simulink model "driver_model_replanning_R1"  (R2023b)
settings: Solver=VariableStepAuto  StartTime=0.0  StopTime=50  RelTol=1e-3
libraries: slpidlib x2, Solver_SF x1
settings Model: DataTypeOverride=Double  MinMaxOverflowLogging=ForceOff  Creator=황수빈  LastModifiedBy=황수빈

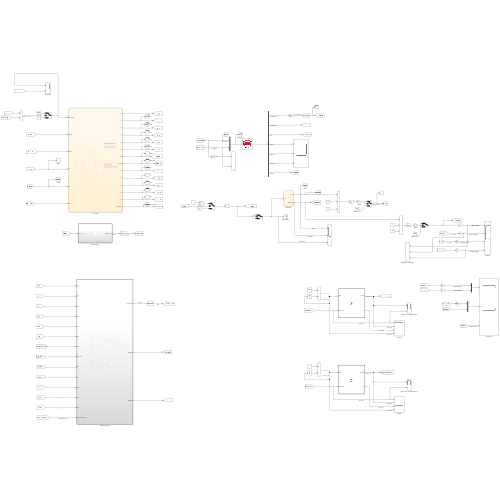
[thumbnail: Simulink's stored preview of the top-level diagram]
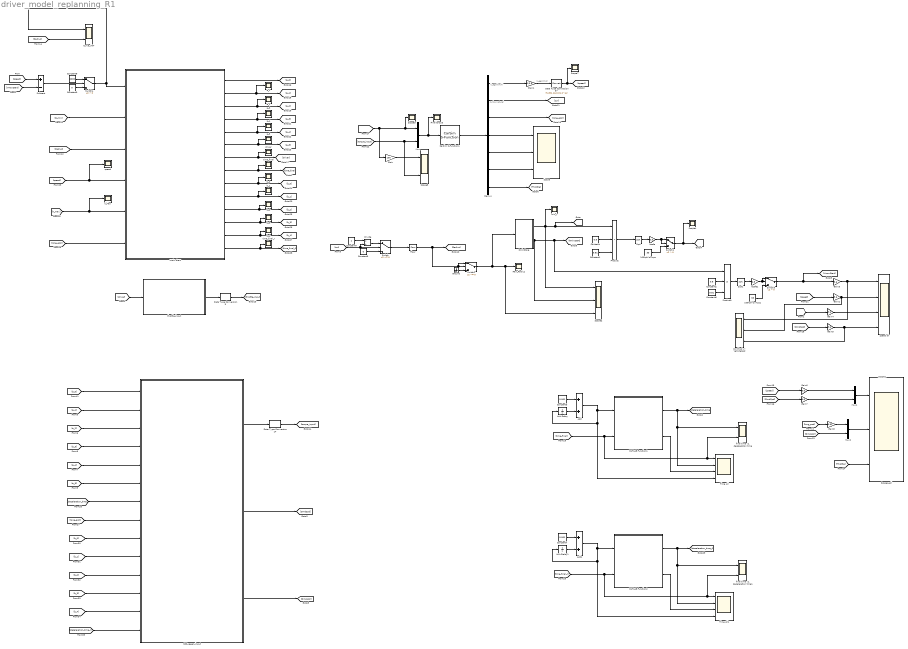
== system driver_model_replanning_R1 ==
  note: V_ego(m/s)
  note: V_ego(km/h)
  note: cur(curvature)
  100kph to mps : Constant  Value=33
  100kph to mps1 : Constant  Value=33
  Add : Sum
  Add1 : Sum
  CarSim S-Function1 : Solver_SF/CarSim S-Function  Priority=1  SIMFILE=simfile.sim  Run_RTs=off  vs_state_ind=Run  StopMode_ind=Vehicle Model
  Constant : Constant  Value=0.8
  Constant1 : Constant  Value=9.81
  Constant2 : Constant  Value=0.8
  Constant3 : Constant  Value=0.001
  Constant4 : Constant
  Constant5 : Constant  Value=0
  Constant6 : Constant  Value=9.81
  Constant7 : Constant  Value=0.001
  Constant8 : Constant  Value=2000
  Constant9 : Constant  Value=0
  Curve_INIT : Scope  NumInputPorts=2
  Data Type Conversion14 : DataTypeConversion  OutDataTypeStr=fixdt(1,16,0)  RndMeth=Nearest  SaturateOnIntegerOverflow=off
  Data Type Conversion3 : DataTypeConversion  OutDataTypeStr=fixdt(1,16,0)  RndMeth=Nearest  SaturateOnIntegerOverflow=off
  Data Type Conversion37 : DataTypeConversion  OutDataTypeStr=fixdt(1,16,0.01,2^-6)  RndMeth=Simplest  SaturateOnIntegerOverflow=off
  Demux : Demux  Outputs=7
  Divide : Product  Inputs=*/
  DmdSpd vs VehicleSpd : Scope  NumInputPorts=3
  Final torque : Scope
  Floor : Rounding
  Gain : Gain  Gain=100
  Gain1 : Gain  Gain=1/3.6
  Gain{2..7} (6 alike) : Gain  Gain=3.6
  Gain8 : Gain  Gain=9.81
  Ground : Ground
  MATLAB Function1 : MATLAB Function  TreatAsAtomicUnit=on
  MATLAB Function2 : MATLAB Function  TreatAsAtomicUnit=on
  Mux : Mux  Inputs=2
  Mux1 : Mux  Inputs=2
  Mux2 : Mux  Inputs=2
  Nsafe : Gain  Gain=0.5
  Nsafe1 : Gain  Gain=0.5
  Product : Product  Inputs=3
  Product1 : Product  Inputs=3
  Raw_Radius : Scope
  RminStore : Stateflow chart  TreatAsAtomicUnit=on
  SRS_regen_input : Subsystem  TreatAsAtomicUnit=on
  Scope : Scope  NumInputPorts=3
  Scope{1,3..4,7} (4 alike) : Scope
  Scope2 : Scope  NumInputPorts=3
  Scope5 : Scope  NumInputPorts=2
  Scopes_all : Scope  NumInputPorts=3
  Sqrt : Sqrt
  Sqrt1 : Sqrt
  Subtract : Sum  Inputs=+-
  Switch : Switch  Criteria=u2 ~= 0  SaturateOnIntegerOverflow=off  InputSameDT=off
  Switch1 : Switch  Criteria=u2 > Threshold  SaturateOnIntegerOverflow=off  InputSameDT=off
  Switch2 : Switch  Criteria=u2 ~= 0  SaturateOnIntegerOverflow=off  InputSameDT=off
  Switch3 : Switch  Criteria=u2 > Threshold  SaturateOnIntegerOverflow=off  InputSameDT=off
  Switch4 : Switch  Criteria=u2 > Threshold  SaturateOnIntegerOverflow=off  InputSameDT=off
  Time All : Scope  NumInputPorts=4
  Time All1 : Scope  NumInputPorts=4
  Unit Delay : UnitDelay  SampleTime=-1  HasFrameUpgradeWarning=on
  Unit Delay1 : UnitDelay  SampleTime=-1  HasFrameUpgradeWarning=on
  V_Max : Scope
  a_{1..5} (5 alike) : Scope
  b_{0..4} (5 alike) : Scope
  driver : Scope
  final time vs. deceleration time : Scope  NumInputPorts=2
  final time vs. deceleration time1 : Scope  NumInputPorts=2
  main chart : Stateflow chart  TreatAsAtomicUnit=on
  min_r : Scope
  speed : Scope
  speed all : Scope  NumInputPorts=4
  throttle_input : Subsystem  TreatAsAtomicUnit=on  SystemSampleTime=0.01
  time_final : Scope
  time_final_r : Scope
  wires:
  [a_4] -> SRS_regen_input/5(a_4)
  [speed] -> Gain2/1  "m/s -> kph"
  100kph to mps/1 -> Switch1/3
  [a_3] -> SRS_regen_input/4(a_3)
  Gain/1 -> Scope5/1
  [Throttle] -> Scopes_all/3  "Throttle Pressure"
  Gain7/1 -> Mux1/2  "TARGET SPEED"
  Floor/1 -> Switch2/1, Switch2/2, [Radius]
  [DmdSpd] -> Gain7/1
  [DmdAccl] -> Mux2/2
  Sqrt1/1 -> Nsafe1/1
  [deceleration_time] -> SRS_regen_input/7(time t)
  Gain6/1 -> Mux1/1  "VEHICLE SPEED"
  Mux2/1 -> Scopes_all/2
  Demux/2 -> [cur]
  Product1/1 -> Sqrt1/1
  Gain8/1 -> Mux2/1
  Gain5/1 -> DmdSpd vs VehicleSpd/3, speed all/4  "DEMAND SPEED"
  Mux1/1 -> Scopes_all/1
  Add/1 -> Unit Delay/1, Time All/4, MATLAB Function1/1(time)  "current_time"
  [long_accl] -> Gain8/1
  Demux/5 -> Scope/2  "M_Mtr_D2"
  Demux/7 -> [Throttle]  "Thrtl_SC"
  Nsafe/1 -> Switch1/1, Switch1/2
  SRS_regen_input/3(DmdAccl) -> [DmdAccl]
  [speed] -> Gain6/1
  SRS_regen_input/2(DmdSpd) -> [DmdSpd]
  Switch3/1 -> [VmaxStart], Gain3/1
  100kph to mps1/1 -> Switch3/3
  MATLAB Function1/1(t_output) -> [deceleration_time], final time vs. deceleration time/1, Time All/2  "decel_time"
  [Radius] -> main chart/3(radius)
  main chart/4(a_3) -> a_3/1, [a_3]
  [DmdSpd] -> Gain5/1
  Demux/6 -> Scope/3  "PwMtC_D2"
  [V_max] -> Gain4/1  "m/s -> kph"
  [a_2] -> SRS_regen_input/3(a_2)
  Demux/1 -> Gain1/1
  Gain4/1 -> speed all/3  "TARGET SPEED2"
  Constant2/1 -> Product1/2
  Unit Delay/1 -> Add/2
  Demux/4 -> Scope/1  "M_Mt_D2"
  Gain3/1 -> DmdSpd vs VehicleSpd/1, speed all/1  "TARGET SPEED"
  Nsafe1/1 -> Switch3/1, Switch3/2
  [Radius] -> Curve_INIT/2
  Product/1 -> Sqrt/1
  main chart/5(a_4) -> [a_4], a_4/1
  [speed] -> speed/1, main chart/4(v0)
  RminStore/1(Rmin) -> min_r/1, [R_min], Product/1, Scope2/1  "minR"
  Switch2/1 -> Scope2/3, Raw_Radius/1, RminStore/1(r)  "Raw Radius"
  [long_accl] -> SRS_regen_input/8(long. accl)
  [throttle_input] -> Mux/1, Scope3/1, Gain/1  "throttle input"
  Sqrt/1 -> Nsafe/1
  [torque_input] -> Scope5/2, Mux/2  "torque input"
  Ground/1 -> Switch2/3
  Gain1/1 -> Data Type Conversion37/1
  [a_5] -> SRS_regen_input/6(a_5)
  [time_final] -> MATLAB Function1/2(time_final), final time vs. deceleration time/2, Time All/1  "time_final"
  [long_accl] -> main chart/6(a0)
  [R_min] -> main chart/2(R_min)
  Constant3/1 -> Add/1
  Constant9/1 -> Switch4/3
  throttle_input/1(throttle_input) -> Data Type Conversion3/1  "before"
  Constant/1 -> Product/2
  Switch4/1 -> main chart/1(Curve_INIT), Curve_INIT/1
  Subtract/1 -> Switch4/2  "speed > v_max"
  [V_max] -> V_Max/1, main chart/5(vf)
  MATLAB Function1/2(p) -> Time All/3  "prev_time"
  [VmaxStart] -> Subtract/2
  [a_1] -> SRS_regen_input/2(a_1)
  main chart/2(a_1) -> a_1/1, [a_1]
  main chart/3(a_2) -> a_2/1, [a_2]
  main chart/6(a_5) -> [a_5], a_5/1
  [a_0] -> SRS_regen_input/1(a_0)
  Constant8/1 -> Switch4/1
  Mux/1 -> CarSim S-Function1/1, Final torque/1
  Data Type Conversion3/1 -> [throttle_input]  "after"
  main chart/7(driver) -> [driver], driver/1
  Data Type Conversion37/1 -> Scope7/1, [speed]
  Demux/3 -> [long_accl]  "accel"
  Divide/1 -> Switch/1
  [cur] -> Switch/2, Divide/2
  RminStore/2(RminStart) -> Scope2/2, [RminStart], Product1/1  "minR Start"
  main chart/8(time_final) -> [time_final], time_final/1
  Switch/1 -> Floor/1
  Gain2/1 -> DmdSpd vs VehicleSpd/2, speed all/2  "VEHICLE SPEED"
  [driver] -> throttle_input/1(driver)
  main chart/1(a_0) -> [a_0]
  Constant6/1 -> Product1/3
  Constant1/1 -> Product/3
  Constant4/1 -> Divide/1
  Data Type Conversion14/1 -> [torque_input]  "after"
  [speed] -> Subtract/1
  SRS_regen_input/1(torque_input) -> Data Type Conversion14/1  "before"
  Constant5/1 -> Switch/3
  CarSim S-Function1/1 -> Demux/1
  Switch1/1 -> Scope4/1, [V_max]  "target speed(m/s)"
  main chart/9(b_0) -> b_0/1, [b_0]
  main chart/10(b_1) -> b_1/1, [b_1]
  main chart/11(b_2) -> b_2/1, [b_2]
  main chart/12(b_3) -> b_3/1, [b_3]
  main chart/13(b_4) -> b_4/1, [b_4]
  main chart/14(time_final_r) -> time_final_r/1, [time_final_r]
  [b_0] -> SRS_regen_input/9(b_0)
  [b_1] -> SRS_regen_input/10(b_1)
  [b_2] -> SRS_regen_input/11(b_2)
  [b_3] -> SRS_regen_input/12(b_3)  "b_3"
  [b_4] -> SRS_regen_input/13(b_4)  "b_4"
  [time_final_r] -> MATLAB Function2/2(time_final_r), final time vs. deceleration time1/2, Time All1/1  "time_final"
  MATLAB Function2/1(t_output2) -> [deceleration_time_r], final time vs. deceleration time1/1, Time All1/2  "decel_time"
  Unit Delay1/1 -> Add1/2
  Constant7/1 -> Add1/1
  MATLAB Function2/2(p2) -> Time All1/3  "prev_time"
  Add1/1 -> Unit Delay1/1, Time All1/4, MATLAB Function2/1(time)  "current_time"
  [deceleration_time_r] -> SRS_regen_input/14(deceleration_time_r)  "deceleration_time_r"

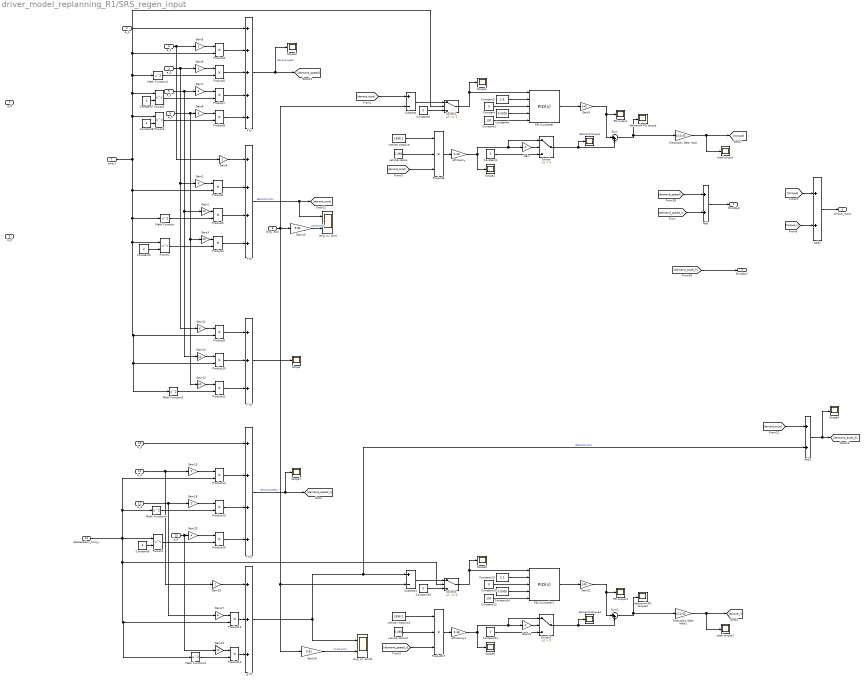
== system driver_model_replanning_R1/SRS_regen_input ==
  a_0 : Inport
  a_1 : Inport  Port=2
  a_2 : Inport  Port=3
  a_3 : Inport  Port=4
  a_4 : Inport  Port=5
  a_5 : Inport  Port=6
  time t : Inport  Port=7
  long. accl : Inport  Port=8
  b_0 : Inport  Port=9
  b_1 : Inport  Port=10
  b_2 : Inport  Port=11
  b_3 : Inport  Port=12
  b_4 : Inport  Port=13
  deceleration_time_r : Inport  Port=14
  Add : Sum
  Add1 : Sum
  Add2 : Sum
  Constant{,1,6,10..11,15} (6 alike) : Constant  Value=0
  Constant12 : Constant  Value=100
  Constant13 : Constant  Value=2.2
  Constant14 : Constant  Value=0.0005
  Constant2 : Constant  Value=100
  Constant3 : Constant  Value=2.8
  Constant4 : Constant  Value=0.0005
  Constant5 : Constant  Value=3
  Constant7 : Constant  Value=3
  Constant8 : Constant  Value=4
  Constant9 : Constant  Value=3
  Gain : Gain  Gain=-1
  Gain1 : Gain  Gain=12
  Gain10 : Gain  Gain=24
  Gain11 : Gain  Gain=6
  Gain12 : Gain  Gain=60
  Gain{4..5,13,19} (4 alike) : Gain  Gain=2
  Gain14 : Gain  Gain=12
  Gain15 : Gain  Gain=9.81
  Gain16 : Gain  Gain=9.81
  Gain17 : Gain  Gain=6
  Gain18 : Gain  Gain=3
  Gain2 : Gain  Gain=6
  Gain20 : Gain  Gain=4
  Gain21 : Gain  Gain=-1
  Gain22 : Gain  Gain=245
  Gain3 : Gain  Gain=20
  Gain6 : Gain  Gain=3
  Gain7 : Gain  Gain=4
  Gain8 : Gain  Gain=5
  Gain9 : Gain  Gain=245
  Math Function{,1..4} (5 alike) : Math  Operator=square
  PD output : Scope
  PD output1 : Scope
  PID Controller : slpidlib/PID Controller  Controller=PID  Form=Parallel  TimeDomain=Continuous-time  UseExternalTs=off  SampleTime=-1  IntegratorMethod=Forward Euler  FilterMethod=Forward Euler  ControllerParametersSource=external  P=1  I=1  UseKiTs=off  D=0  N=100  UseFilter=on  TunerSelectOption=Transfer Function Based (PID Tuner App)  InitialConditionSource=internal  InitialConditionForIntegrator=0  InitialConditionForFilter=0  DifferentiatorICPrevScaledInput=0  ExternalReset=none  TrackingMode=off  Kt=1  LimitOutput=off  SatLimitsSource=internal  UpperSaturationLimit=inf  LowerSaturationLimit=-inf  LinearizeAsGain=on  AntiWindupMode=none  Kb=1  LimitIntegrator=off  UpperIntegratorSaturationLimit=inf  LowerIntegratorSaturationLimit=-inf  POutMin=[]  POutMax=[]  IOutMin=[]  IOutMax=[]  DOutMin=[]  DOutMax=[]  NOutMin=[]  NOutMax=[]  SumOutMin=[]  SumOutMax=[]  SaturationOutMin=[]  SaturationOutMax=[]  PParamMin=[]  PParamMax=[]  IParamMin=[]  IParamMax=[]  DParamMin=[]  DParamMax=[]  NParamMin=[]  NParamMax=[]  KbParamMin=[]  KbParamMax=[]  KtParamMin=[]  KtParamMax=[]  KbOutMin=[]  KbOutMax=[]  KtOutMin=[]  KtOutMax=[]  IntegratorOutMin=[]  IntegratorOutMax=[]  FilterOutMin=[]  FilterOutMax=[]  SumI1OutMin=[]  SumI1OutMax=[]  SumI2OutMin=[]  SumI2OutMax=[]  SumI3OutMin=[]  SumI3OutMax=[]  SumI4OutMin=[]  SumI4OutMax=[]  SumDOutMin=[]  SumDOutMax=[]  DifferentiatorOutMin=[]  DifferentiatorOutMax=[]  FilterDiffOutCoefMin=[]  FilterDiffOutCoefMax=[]  ReciprocalOutMin=[]  ReciprocalOutMax=[]  SumDenOutMin=[]  SumDenOutMax=[]  SumNumOutMin=[]  SumNumOutMax=[]  DivideOutMin=[]  DivideOutMax=[]  UdiffTsProdOutMin=[]  UdiffTsProdOutMax=[]  NTsProdOutMin=[]  NTsProdOutMax=[]  UintegralTsProdOutMin=[]  UintegralTsProdOutMax=[]  UngainTsProdOutMin=[]  UngainTsProdOutMax=[]  ClampingZeroOutDataTypeStr=Inherit: Inherit via back propagation  ClampingZeroOutMin=[]  ClampingZeroOutMax=[]  FilterDenConstantOutDataTypeStr=Inherit: Inherit via back propagation  FilterDenConstantOutMin=[]  FilterDenConstantOutMax=[]  PCopyOutDataTypeStr=Inherit: Inherit via back propagation  PCopyOutMin=[]  PCopyOutMax=[]  NCopyOutDataTypeStr=Inherit: Inherit via back propagation  NCopyOutMin=[]  NCopyOutMax=[]  IntegratorContinuousStateAttributes=''  IntegratorStateMustResolveToSignalObject=off  IntegratorRTWStateStorageClass=Auto  FilterContinuousStateAttributes=''  FilterStateMustResolveToSignalObject=off  FilterRTWStateStorageClass=Auto  ParallelPVariant=ExternalParameters  IdealPVariant=Disabled  IVariant=ExternalParameters  DVariant=ExternalParameters  IntegratorVariant=Continuous  SatVariant=Disabled  AWVariant=Passthrough  PCopyVariant=Disabled  TRVariant=Disabled  FdbkBlocksVariant=Forward  IdealPFdbkVariant=Disabled  SatFdbkVariant=Disabled  DerivativeFilterVariant=ContFilter  NVariant=ExternalParameters  NCopyVariant=Disabled  FilterICVariant=InternalICsFilter  IntegratorICVariant=InternalICs  ExternalResetVariant=Disabled  TRSumVariant=Passthrough  SumFdbkVariant=Disabled  SumVariant=Sum_PID  TsampFilterVariant=InternalTs  TsampNgainVariant=Passthrough  TsampIntegralVariant=Disabled_SignalSpec  ExternalSaturationOutDataTypeStr=Inherit: Same as second input
  PID Controller1 : slpidlib/PID Controller  Controller=PID  Form=Parallel  TimeDomain=Continuous-time  UseExternalTs=off  SampleTime=-1  IntegratorMethod=Forward Euler  FilterMethod=Forward Euler  ControllerParametersSource=external  P=1  I=1  UseKiTs=off  D=0  N=100  UseFilter=on  TunerSelectOption=Transfer Function Based (PID Tuner App)  InitialConditionSource=internal  InitialConditionForIntegrator=0  InitialConditionForFilter=0  DifferentiatorICPrevScaledInput=0  ExternalReset=none  TrackingMode=off  Kt=1  LimitOutput=off  SatLimitsSource=internal  UpperSaturationLimit=inf  LowerSaturationLimit=-inf  LinearizeAsGain=on  AntiWindupMode=none  Kb=1  LimitIntegrator=off  UpperIntegratorSaturationLimit=inf  LowerIntegratorSaturationLimit=-inf  POutMin=[]  POutMax=[]  IOutMin=[]  IOutMax=[]  DOutMin=[]  DOutMax=[]  NOutMin=[]  NOutMax=[]  SumOutMin=[]  SumOutMax=[]  SaturationOutMin=[]  SaturationOutMax=[]  PParamMin=[]  PParamMax=[]  IParamMin=[]  IParamMax=[]  DParamMin=[]  DParamMax=[]  NParamMin=[]  NParamMax=[]  KbParamMin=[]  KbParamMax=[]  KtParamMin=[]  KtParamMax=[]  KbOutMin=[]  KbOutMax=[]  KtOutMin=[]  KtOutMax=[]  IntegratorOutMin=[]  IntegratorOutMax=[]  FilterOutMin=[]  FilterOutMax=[]  SumI1OutMin=[]  SumI1OutMax=[]  SumI2OutMin=[]  SumI2OutMax=[]  SumI3OutMin=[]  SumI3OutMax=[]  SumI4OutMin=[]  SumI4OutMax=[]  SumDOutMin=[]  SumDOutMax=[]  DifferentiatorOutMin=[]  DifferentiatorOutMax=[]  FilterDiffOutCoefMin=[]  FilterDiffOutCoefMax=[]  ReciprocalOutMin=[]  ReciprocalOutMax=[]  SumDenOutMin=[]  SumDenOutMax=[]  SumNumOutMin=[]  SumNumOutMax=[]  DivideOutMin=[]  DivideOutMax=[]  UdiffTsProdOutMin=[]  UdiffTsProdOutMax=[]  NTsProdOutMin=[]  NTsProdOutMax=[]  UintegralTsProdOutMin=[]  UintegralTsProdOutMax=[]  UngainTsProdOutMin=[]  UngainTsProdOutMax=[]  ClampingZeroOutDataTypeStr=Inherit: Inherit via back propagation  ClampingZeroOutMin=[]  ClampingZeroOutMax=[]  FilterDenConstantOutDataTypeStr=Inherit: Inherit via back propagation  FilterDenConstantOutMin=[]  FilterDenConstantOutMax=[]  PCopyOutDataTypeStr=Inherit: Inherit via back propagation  PCopyOutMin=[]  PCopyOutMax=[]  NCopyOutDataTypeStr=Inherit: Inherit via back propagation  NCopyOutMin=[]  NCopyOutMax=[]  IntegratorContinuousStateAttributes=''  IntegratorStateMustResolveToSignalObject=off  IntegratorRTWStateStorageClass=Auto  FilterContinuousStateAttributes=''  FilterStateMustResolveToSignalObject=off  FilterRTWStateStorageClass=Auto  ParallelPVariant=ExternalParameters  IdealPVariant=Disabled  IVariant=ExternalParameters  DVariant=ExternalParameters  IntegratorVariant=Continuous  SatVariant=Disabled  AWVariant=Passthrough  PCopyVariant=Disabled  TRVariant=Disabled  FdbkBlocksVariant=Forward  IdealPFdbkVariant=Disabled  SatFdbkVariant=Disabled  DerivativeFilterVariant=ContFilter  NVariant=ExternalParameters  NCopyVariant=Disabled  FilterICVariant=InternalICsFilter  IntegratorICVariant=InternalICs  ExternalResetVariant=Disabled  TRSumVariant=Passthrough  SumFdbkVariant=Disabled  SumVariant=Sum_PID  TsampFilterVariant=InternalTs  TsampNgainVariant=Passthrough  TsampIntegralVariant=Disabled_SignalSpec  ExternalSaturationOutDataTypeStr=Inherit: Same as second input
  Power{1..4} (4 alike) : Math  Operator=pow
  Product{1..5,7..16} (15 alike) : Product
  Product17 : Product  Inputs=3
  Product6 : Product  Inputs=3
  Reduction Gear ratio : Gain  Gain=1/10.65
  Reduction Gear ratio1 : Gain  Gain=1/10.65
  Scope{,1..7} (8 alike) : Scope
  Subtract : Sum  Inputs=+-
  Subtract1 : Sum  Inputs=+-
  Sum : Sum  Inputs=|++
  Sum1 : Sum  Inputs=|++
  Switch : Switch  Criteria=u2 > Threshold  SaturateOnIntegerOverflow=off  InputSameDT=off
  Switch1 : Switch  Criteria=u2 ~= 0  SaturateOnIntegerOverflow=off  InputSameDT=off
  Switch2 : Switch  Criteria=u2 > Threshold  SaturateOnIntegerOverflow=off  InputSameDT=off
  Switch3 : Switch  Criteria=u2 ~= 0  SaturateOnIntegerOverflow=off  InputSameDT=off
  demand torque : Scope
  demand torque1 : Scope
  demand+PD torque : Scope
  demand+PD torque1 : Scope
  efficiency : Gain  Gain=0.46
  efficiency1 : Gain  Gain=0.46
  f'''(t) : Sum  Inputs=+++
  f''(t) : Sum  Inputs=4
  f'(t) : Sum  Inputs=5
  f'(t)1 : Sum  Inputs=4
  g''(t) : Sum  Inputs=3
  long vs. dmd : Scope  NumInputPorts=2
  long vs. dmd1 : Scope  NumInputPorts=2
  total torque : Scope
  total torque1 : Scope
  vehicle massive : Constant  Value=1898.2
  vehicle massive1 : Constant  Value=1898.2
  vehicle radius : Constant  Value=0.468
  vehicle radius1 : Constant  Value=0.468
  torque_input : Outport
  DmdSpd : Outport  Port=2
  DmdAccl : Outport  Port=3
  wires:
  Constant5/1 -> Power1/2
  Product2/1 -> f''(t)/3
  Product4/1 -> f''(t)/4
  Power1/1 -> Product4/2
  Math Function/1 -> Product2/2
  Product6/1 -> efficiency/1
  efficiency/1 -> Scope2/1, Switch/1, Gain/1
  Constant1/1 -> Switch/3
  Gain/1 -> Switch/2
  f''(t)/1 -> long vs. dmd/1, [demand_accel]  "DEMAND ACCL"
  Gain1/1 -> Product2/1
  Gain3/1 -> Product4/1
  Gain4/1 -> f''(t)/1
  Gain2/1 -> Product1/1
  Product1/1 -> f''(t)/2
  Subtract/1 -> Switch1/1
  Switch1/1 -> PID Controller/1, Scope1/1
  Constant6/1 -> Switch1/3
  Constant2/1 -> PID Controller/5
  Constant4/1 -> PID Controller/4
  Constant/1 -> PID Controller/3
  Constant3/1 -> PID Controller/2
  PID Controller/1 -> Gain9/1
  Product3/1 -> f'(t)/2
  Product5/1 -> f'(t)/3
  Product7/1 -> f'(t)/4
  Product8/1 -> f'(t)/5
  Gain5/1 -> Product3/1
  Gain6/1 -> Product5/1
  Gain7/1 -> Product7/1
  Gain8/1 -> Product8/1
  f'(t)/1 -> Scope3/1, [demand_speed]  "demand speed"
  Math Function1/1 -> Product5/2
  Power2/1 -> Product7/2
  Power3/1 -> Product8/2
  Constant7/1 -> Power2/2
  Constant8/1 -> Power3/2
  Switch/1 -> Sum/2, demand torque/1
  Gain15/1 -> long vs. dmd/2  "LONG.ACCL"
  vehicle radius/1 -> Product6/2
  vehicle massive/1 -> Product6/1
  Sum/1 -> Reduction Gear ratio/1, demand+PD torque/1
  Gain9/1 -> PD output/1, Sum/1
  Reduction Gear ratio/1 -> [torque], total torque/1
  Gain12/1 -> Product11/1
  Gain10/1 -> Product10/1
  Gain11/1 -> Product9/1
  a_1/1 -> f'(t)/1
  a_2/1 -> Gain5/1, Gain4/1
  a_3/1 -> Gain11/1, Gain2/1, Gain6/1
  a_4/1 -> Gain10/1, Gain1/1, Gain7/1
  a_5/1 -> Gain3/1, Gain12/1, Gain8/1
  Math Function2/1 -> Product11/2
  time t/1 -> Power1/1, Product9/2, Product10/2, Math Function2/1, Math Function/1, Product1/2, Switch1/2, Product3/2, Math Function1/1, Power2/1, Power3/1
  Product9/1 -> f'''(t)/1
  Product10/1 -> f'''(t)/2
  Product11/1 -> f'''(t)/3
  f'''(t)/1 -> Scope/1
  b_2/1 -> Gain19/1, Gain13/1
  g''(t)/1 -> Add1/2, Subtract1/1, long vs. dmd1/1  "DEMAND ACCL"
  Gain14/1 -> Product13/1
  Gain19/1 -> g''(t)/1
  Gain16/1 -> long vs. dmd1/2  "LONG.ACCL"
  Product12/1 -> g''(t)/2
  Gain17/1 -> Product12/1
  Product13/1 -> g''(t)/3
  Math Function3/1 -> Product13/2
  b_4/1 -> Gain14/1, Gain20/1
  b_3/1 -> Gain18/1, Gain17/1
  [demand_accel] -> Subtract/1
  long. accl/1 -> Subtract/2, Gain16/1, Subtract1/2, Gain15/1
  [demand_accel] -> Product6/3
  [demand_accel] -> Add1/1
  Add1/1 -> Scope4/1, [demand_accel_S]
  b_1/1 -> f'(t)1/1
  deceleration_time_r/1 -> Math Function3/1, Product12/2, Switch3/2, Product14/2, Math Function4/1, Power4/1
  Constant9/1 -> Power4/2
  f'(t)1/1 -> Scope7/1, [demand_speed_r]  "demand speed_r"
  Power4/1 -> Product16/2
  Gain13/1 -> Product14/1
  Product14/1 -> f'(t)1/2
  Gain18/1 -> Product15/1
  Gain20/1 -> Product16/1
  Math Function4/1 -> Product15/2
  Product16/1 -> f'(t)1/4
  Product15/1 -> f'(t)1/3
  [demand_speed] -> Add/1
  [demand_speed_r] -> Add/2
  Add/1 -> DmdSpd/1
  [demand_accel_S] -> DmdAccl/1
  [demand_speed_r] -> Product17/3
  Switch2/1 -> Sum1/2, demand torque1/1
  efficiency1/1 -> Scope6/1, Switch2/1, Gain21/1
  Gain22/1 -> PD output1/1, Sum1/1
  Constant12/1 -> PID Controller1/5
  vehicle radius1/1 -> Product17/2
  Constant15/1 -> Switch3/3
  Reduction Gear ratio1/1 -> [torque_r], total torque1/1
  Sum1/1 -> Reduction Gear ratio1/1, demand+PD torque1/1
  PID Controller1/1 -> Gain22/1
  vehicle massive1/1 -> Product17/1
  Constant10/1 -> PID Controller1/3
  Constant14/1 -> PID Controller1/4
  Switch3/1 -> PID Controller1/1, Scope5/1
  Constant13/1 -> PID Controller1/2
  Subtract1/1 -> Switch3/1
  Gain21/1 -> Switch2/2
  Product17/1 -> efficiency1/1
  Constant11/1 -> Switch2/3
  [torque] -> Add2/1
  [torque_r] -> Add2/2
  Add2/1 -> torque_input/1

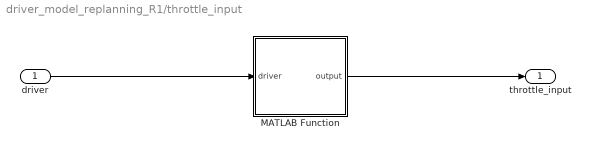
== system driver_model_replanning_R1/throttle_input ==
  driver : Inport
  MATLAB Function : MATLAB Function  TreatAsAtomicUnit=on
  throttle_input : Outport
  wires:
  driver/1 -> MATLAB Function/1(driver)
  MATLAB Function/1(output) -> throttle_input/1

== stateflow chart driver_model_replanning_R1/main chart ==
  state CurveRoadState
    during:
    driver = 0;
    if (radius-2500 == R_min )
    if v0 ~= 0
    if (flag_v == 0)
    vv = v0;
    flag_v = 1;
    end
    end
    a_min = -3;
    t_margin = 0.1;
    [time_final, time_final_r, distance_r] = var_cal(v0, vf, a_min, t_margin);
    if distance ~= 0
    dd = distance;
    end
    if time_final ~= 0
    tt = time_final;
    end
    if v0 ~= 0
    if (flag_a == 0)
    aa = a0;
    flag_a = 1;
    end
    end
    [a_0, a_1, a_2, a_3, a_4, a_5] = calculate(v0, a0, vf, distance, time_final, distance_r, time_final_r);
    else
    flag_v = 0;
    flag_a = 0;
    end
  state InitialState
    driver = 0;
    time_final=0;
    time_final_r=0;
    aa = 0;
    vv = 0;
    dd = 0;
    tt = 0;
    dd_r = 0;
    tt_r = 0;
    vv_r = 0;
    flag_v = 0;
    flag_a = 0;
    am = 0;
  state KeepSpdState
    driver = 2;
    distance_r = 0;
    time_final_r = 0;
    tt_r=0;
    vv=0;
    dd_r=0;
    am = 0;
    b_0=0;
    b_1=0;
    b_2=0;
    b_3=0;
    b_4=0;
  state PowerAccelState
    driver = 3;
  state NormAccelState
    driver = 1;
  (default) -> InitialState
  CurveRoadState -> (junction 83) : [Curve_INIT==0]
  InitialState -> CurveRoadState [order 1] : [Curve_INIT ~= 0 ]
  (junction 83) -> KeepSpdState
  (junction 87) -> CurveRoadState
  PowerAccelState -> (junction 87) : [Curve_INIT ~= 0]
  InitialState -> (junction 46) [order 2] : [Curve_INIT==0]
  (junction 46) -> PowerAccelState
  KeepSpdState -> (junction 85) : [radius > R_min]
  (junction 85) -> NormAccelState
  NormAccelState -> (junction 163) : [Curve_INIT ==0]
  (junction 163) -> (junction 164)
  (junction 164) -> NormAccelState
  data: time_final function_output; time_final_r function_output; v0 function_input; vf function_input; a_min function_input; t_margin function_input; distance_r function_output; a_0 function_output; v0 function_input; a0 function_input; vf function_input; a_1 function_output; a_2 function_output; a_3 function_output; a_4 function_output; a_5 function_output; distance function_input; time_final function_input; distance_r function_input; time_final_r function_input; Curve_INIT input; R_min input; radius input; v0 input; vf input; a_0 output; a_1 output; a_2 output; a_3 output; a_4 output; a_5 output; driver output; time_final output; tt local; aa local; dd local; distance local; a0 input; flag_v local; flag_a local; vv local; b_0 output; b_1 output; b_2 output; b_3 output; b_4 output; time_final_r output; distance_r local; vv_r local; tt_r local; dd_r local; am local; t1 local; t2 local; a_min local; t_margin local
  function [time_final, time_final_r, distance_r] = var_cal(v0, vf, a_min, t_margin):
    | function [time_final, time_final_r, distance_r] = var_cal(v0, vf, a_min, t_margin)
    |     % radius: 입력 값
    |     % v0: 초기 속도
    |     % vf: 최종 속도
    |     % distance: 조건에 따른 결과 값
    |     % tf: 계산된 시간 (distance / ((v0 + vf) / 2))
    | 
    |     %a_target = (a0 + 0) / 2;
    | 
    |     % 조건에 따라 distance 설정
    |     if R_min == 56
    |         distance = 266.5;
    |     elseif R_min == 108
    |         distance = 80;
    |     elseif R_min == 220
    |         distance = 138.5;
    |             % 기본 값 설정
    |     else
    |             distance = NaN;  % 유효한 값이 없을 때 NaN 반환
    |     end
    |     
    |     % tf 계산 (distance가 NaN이 아니면 계산)
    |     if ~isnan(distance)
    |         %a_final = a_target + a_slope;
    |         %time_final = (vf - v0) / a_final;
    |         time_final = distance / ((v0 + vf) / 2);  % 평균 속도를 사용하여 시간 계산
    |     else
    |         time_final = NaN;  % distance가 유효하지 않으면 tf도 NaN으로 설정
    |     end
    |      %% constraint 고려했을 때
    | 
    |     % -3 < 3(vf - v0)/(2*tf) 를 만족하는 최소 tf 계산
    |     numerator = 3 * (vf - v0);
    |     denominator = 2 * a_min;
    | 
    |     % 계산된 tf 경계값
    |     tf_candidate = numerator / denominator;
    |     
    |     %tf는 양수여야 하므로 0보다 작으면 무의미
    |     if tf_candidate <= 0
    |         time_final_r = NaN;  % 또는 예외 처리
    |         distance_r = NaN;
    |         return;
    |     end
    | 
    |     % replanning tf_r 계산
    |     time_final_r = ceil(tf_candidate * 10) / 10 + t_margin;
    |     distance_r = time_final_r * (v0 + vf) / 2;
    | end
  function [a_0, a_1, a_2, a_3, a_4, a_5] =  calculate(v0, a0, vf, distance, time_final, distance_r, time_final_r):
    | function [a_0, a_1, a_2, a_3, a_4, a_5] =  calculate(v0, a0, vf, distance, time_final, distance_r, time_final_r)
    | 
    | a_0 = 0;
    | 
    | %% 5차 profiling %%
    | xf = distance;
    | tf = time_final;
    | af = 0; %임의로 지정
    | 
    | P = [1, 0, 0, 0, 0, 0;
    |     0, 1, 0, 0, 0, 0;
    |     0, 0, 2, 0, 0, 0;
    |     1, tf, tf^2, tf^3, tf^4, tf^5;
    |     0, 1, 2*tf, 3*tf^2, 4*tf^3, 5*tf^4;
    |     0, 0, 2, 6*tf, 12*tf^2, 20*tf^3;];
    | 
    | Q = [0; v0; a0; xf; vf; af;];
    | 
    | % 연립 방정식 풀기 (A \ B 사용)
    | coeffs = P \ Q;
    | 
    | % 계수 추출 (초기 계산에서의 계수는 b로 칭함)
    | b_1 = coeffs(2);
    | b_2 = coeffs(3);
    | b_3 = coeffs(4);
    | b_4 = coeffs(5);
    | b_5 = coeffs(6);
    | 
    | %% solve Jerk Root: j(t) = 6*b3 + 24*b4*t + 60*b5*t^2 = 0 의 해 계산 %%
    | % 입력: b3, b4, b5
    | % 출력: t1, t2 (두 개의 실근 또는 복소수근 반환)
    | 
    | % 계수 설정 (표준 2차형식 At^2 + Bt + C)
    | A = 60 * b_5;
    | B = 24 * b_4;
    | C = 6  * b_3;
    | 
    | % 판별식 계산
    | D = B^2 - 4*A*C;
    | 
    | % 해 계산
    | if A == 0
    | % 선형 방정식으로 처리 (예외 처리)
    |     if B ~= 0
    |         t1 = -C / B;
    |         t2 = NaN;  % 두 번째 해 없음
    |     else
    |         t1 = NaN;
    |         t2 = NaN;
    |     end
    | else
    |     sqrtD = sqrt(D);  % D < 0이면 복소수 처리됨
    |     t1 = (-B - sqrtD) / (2*A);
    |     t2 = (-B + sqrtD) / (2*A);
    | end
    | % minAcceleration: 두 시간점에서의 가속도를 계산해 더 작은 값 반환
    | 
    | % 각 시간점에서의 가속도 계산
    | a_t1 = 2 * b_2 + 6 * b_3 * t1 + 12 * b_4 * t1^2 + 20 * b_5 * t1^3;
    | a_t2 = 2 * b_2 + 6 * b_3 * t2 + 12 * b_4 * t2^2 + 20 * b_5 * t2^3;
    | 
    | % 둘 다 유효한 숫자인 경우
    | if ~isnan(a_t1) && ~isnan(a_t2)
    |     a_min_ref = min(a_t1, a_t2);
    | 
    | % 하나만 유효한 경우
    | elseif ~isnan(a_t1)
    |     a_min_ref = a_t1;
    | elseif ~isnan(a_t2)
    |     a_min_ref = a_t2;
    | 
    | % 둘 다 유효하지 않은 경우
    | else
    |     a_min_ref = NaN;
    | end
    | 
    | 
    | %% 임계값을 넘어가면 constraint를 고려하여 계수 재계산 및 확정 %%
    | if a_min_ref <= -3
    |     xf = distance_r;
    |     tf = time_final_r;
    |     
    |     R = [1, 0, 0, 0, 0;
    |     0, 1, 0, 0, 0;
    |     0, 0, 2, 0, 0;
    |     1, tf, tf^2, tf^3, tf^4;
    |     0, 1, 2*tf, 3*tf^2, 4*tf^3;
    |     0, 0, 2, 6*tf, 12*tf^2;];
    |     
    |     S = [0; v0; 0; xf; vf; 0;]; % a0=0, af=0
    | 
    |     % 연립 방정식 풀기 (R \ S 사용)
    |     coeffs_r = R \ S;
    | 
    |     % 계수 추출
    |     a_1 = coeffs_r(2);
    |     a_2 = coeffs_r(3);
    |     a_3 = coeffs_r(4);
    |     a_4 = coeffs_r(5);
    |     a_5 = coeffs_r(6);
    | else
    |     a_1 = b_1;
    |     a_2 = b_2;
    |     a_3 = b_3;
    |     a_4 = b_4;
    |     a_5 = b_5;
    | end

== matlab function driver_model_replanning_R1/MATLAB Function2 ==
  data: time input; t_output2 output; time_final_r input; p2 output
function [t_output2, p2] = fcn2(time, time_final_r)
    persistent prev_time2;  % 이전 시간 저장용 변수
    if isempty(prev_time2)
        prev_time2 = time;  % 초기화, 첫 호출 시 현재 시간으로 설정
    end

    % time이 time_final에 도달하면 prev_time을 초기화
    if (time - prev_time2) < time_final_r 
        t_output2 = (time - prev_time2);  % time_final에 도달하기 전까지의 값
        p2 = prev_time2;

    
    elseif (time - prev_time2) == time_final_r 
        t_output2 = 0;  % time_final에 도달하기 전까지의 값
        p2 = prev_time2;

    else
        prev_time2 = time;  % 새로운 loop 시작 (time_final 도달 후 초기화)
        t_output2 = 0;  % time_final 도달 후 초기화된 slow_time
        p2 = prev_time2;

    end

end

== matlab function driver_model_replanning_R1/MATLAB Function1 ==
  data: time input; t_output output; time_final input; p output
function [t_output, p] = fcn(time, time_final)
    persistent prev_time;  % 이전 시간 저장용 변수
    if isempty(prev_time)
        prev_time = time;  % 초기화, 첫 호출 시 현재 시간으로 설정
    end

    % time이 time_final에 도달하면 prev_time을 초기화
    if (time - prev_time) < time_final 
        t_output = (time - prev_time);  % time_final에 도달하기 전까지의 값
        p = prev_time;

    
    elseif (time - prev_time) == time_final 
        t_output = 0;  % time_final에 도달하기 전까지의 값
        p = prev_time;

    else
        prev_time = time;  % 새로운 loop 시작 (time_final 도달 후 초기화)
        t_output = 0;  % time_final 도달 후 초기화된 slow_time
        p = prev_time;

    end

end

== matlab function driver_model_replanning_R1/throttle_input/MATLAB Function ==
  data: driver input; output output
function output = driver_function(driver)
    switch driver
        case 0
            output = 0;
        case 1
            output = 0.4;
        case 2
            output = 0.04;
        otherwise
            output = 0.4;
    end
end

== stateflow chart driver_model_replanning_R1/RminStore ==
  state RminStopStoring
    Rmin = minimum;
    RminStart = 0;
  state RminStoring
    if r>2500 && r<3000
    minimum = r-2500;
    end
    Rmin = minimum;
    RminStart = minimum;
  state INITIAL
    minimum = 0;
    Rmin=0;
    RminStart=0;
  (default) -> INITIAL
  INITIAL -> RminStoring : [r > 2500 && r < 3000]
  RminStoring -> RminStopStoring : [minimum == r]
  (junction 19) -> INITIAL
  RminStopStoring -> (junction 14) : [minimum < r]
  (junction 14) -> (junction 19)
  data: r input; Rmin output; minimum local; RminStart output
